simulink model "m03_model_for_HInf"  (R2021a)
settings: Solver=VariableStepAuto  StartTime=0.0  StopTime=20  MaxStep=1e-3  RelTol=1e-3
PreLoadFcn:
  | load feedforward_controller
InitFcn:
  | load feedforward_controller
libraries: cstblocks x3, acolibjan22 x3
settings Model: Creator=e102261  LastModifiedBy=jason
settings SolverCC: AlgebraicLoopSolver=TrustRegion
settings DataIOCC: SaveOutput=off  SignalLogging=off  DSMLogging=off  SaveTime=off  ReturnWorkspaceOutputs=off
settings DebuggingCC: ArithmeticOperatorsInVariantConditions=warning
settings SFSimCC: CustomCodeUndefinedFunction=UseInterfaceOnly

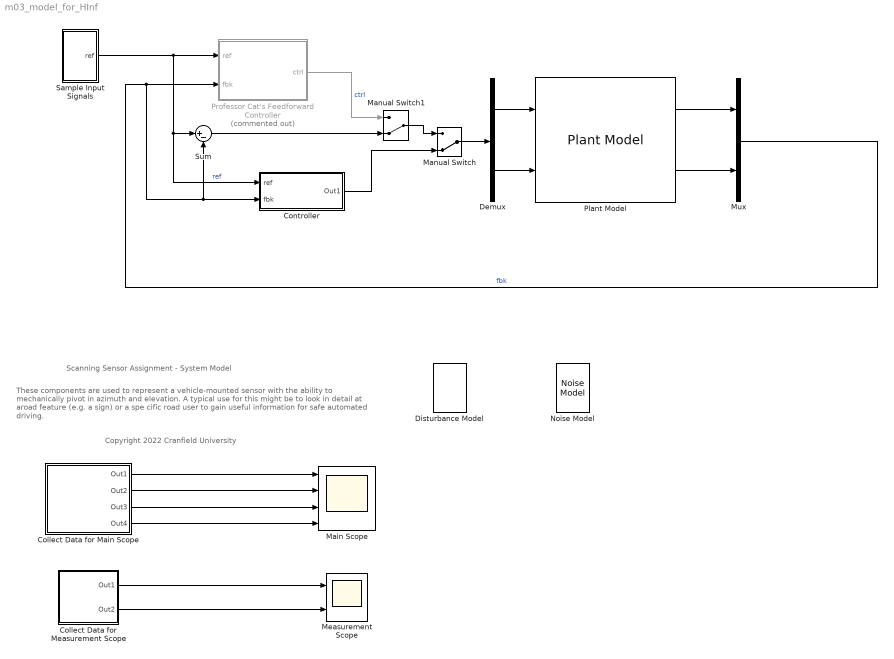
== system m03_model_for_HInf ==
  note: These components are used to represent a vehicle-mounted sensor with the ability to mechanically pivot in azimuth and elevation.  A typical use for this might be to look in
      | detail at aroad feature (e.g. a sign) or a spe cific road user to gain useful information for
      | safe automated driving.
  note: Scanning Sensor Assignment - System Model
  note: Copyright 2022 Cranfield University
  Collect Data for Main Scope : Subsystem
  Collect Data for Measurement Scope : Subsystem
  Controller : Subsystem
  Demux : Demux  Outputs=2
  Disturbance Model : acolibjan22/Disturbance Model  EnabledState=on
      settings: AttributesFormatString=|
      | Your control system is expected to
      | work with this enabled, but it is
      | sometimes helpful to turn it off for
      | debugging.
  Main Scope : Scope  NumInputPorts=4
  Manual Switch : ManualSwitch  CurrentSetting=0
  Manual Switch1 : ManualSwitch  CurrentSetting=0
  Measurement Scope : Scope  NumInputPorts=2
      settings: AttributesFormatString=|
      | There is nothing feedback control
      | can do to make these signals less
      | noisy, but you can reduce the amount
      | of this noise that gets fed back into
      | the control signals.
  Mux : Mux  Inputs=2
  Noise Model : acolibjan22/Noise Model  EnabledState=on
      settings: AttributesFormatString=|
      | Your control system is expected to
      | work with this enabled, but it is
      | sometimes helpful to turn it off for
      | debugging.
  Plant Model : acolibjan22/Plant Model  X0=0
  Professor Cat's Feedforward Controller : Subsystem  Commented=on  LoadFcn=load feedforward_controller  InitFcn=load feedforward_controller
      settings: AttributesFormatString=Your controller replaces this!
      mask Display: image('graphic1.jpg')
  Sample Input Signals : Subsystem
  Sum : Sum  Inputs=|+-
  wires:
  Plant Model/1 -> Mux/1
  Collect Data for Main Scope/1(Out1) -> Main Scope/1
  Collect Data for Main Scope/2(Out2) -> Main Scope/2
  Collect Data for Main Scope/3(Out3) -> Main Scope/3
  Collect Data for Main Scope/4(Out4) -> Main Scope/4
  Mux/1 -> Controller/2(fbk), Sum/2, Professor Cat's Feedforward Controller/2(fbk)  "fbk"
  Plant Model/2 -> Mux/2
  Demux/2 -> Plant Model/2
  Demux/1 -> Plant Model/1
  Collect Data for Measurement Scope/1(Out1) -> Measurement Scope/1
  Collect Data for Measurement Scope/2(Out2) -> Measurement Scope/2
  Sample Input Signals/1(ref) -> Sum/1, Controller/1(ref), Professor Cat's Feedforward Controller/1(ref)  "ref"
  Professor Cat's Feedforward Controller/1(ctrl) -> Manual Switch1/1  "ctrl"
  Manual Switch/1 -> Demux/1
  Controller/1(Out1) -> Manual Switch/2
  Sum/1 -> Manual Switch1/2
  Manual Switch1/1 -> Manual Switch/1

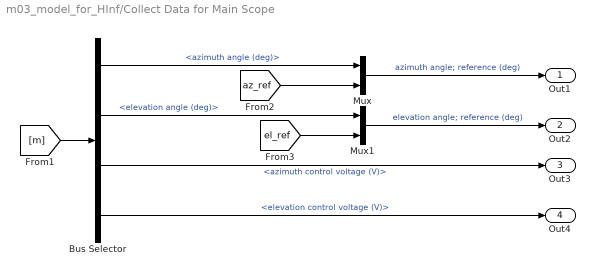
== system m03_model_for_HInf/Collect Data for Main Scope ==
  Bus Selector : BusSelector  OutputSignals=azimuth angle (deg),elevation angle (deg),azimuth control voltage (V),elevation control voltage (V)
  Mux : Mux  Inputs=2
  Mux1 : Mux  Inputs=2
  Out1 : Outport
  Out2 : Outport  Port=2
  Out3 : Outport  Port=3
  Out4 : Outport  Port=4
  wires:
  [m] -> Bus Selector/1
  Mux/1 -> Out1/1  "azimuth angle; reference (deg)"
  Bus Selector/1 -> Mux/1  "<azimuth angle (deg)>"
  [az_ref] -> Mux/2
  Bus Selector/2 -> Mux1/1  "<elevation angle (deg)>"
  [el_ref] -> Mux1/2
  Mux1/1 -> Out2/1  "elevation angle; reference (deg)"
  Bus Selector/3 -> Out3/1  "<azimuth control voltage (V)>"
  Bus Selector/4 -> Out4/1  "<elevation control voltage (V)>"

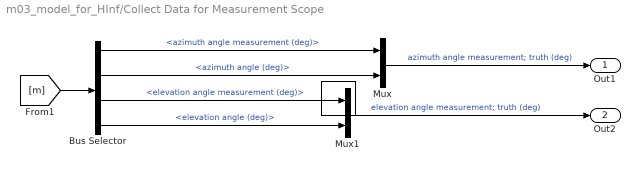
== system m03_model_for_HInf/Collect Data for Measurement Scope ==
  Bus Selector : BusSelector  OutputSignals=azimuth angle measurement (deg),azimuth angle (deg),elevation angle measurement (deg),elevation angle (deg)
  Mux : Mux  Inputs=2
  Mux1 : Mux  Inputs=2
  Out1 : Outport
  Out2 : Outport  Port=2
  wires:
  Mux1/1 -> Out2/1  "elevation angle measurement; truth (deg)"
  Bus Selector/4 -> Mux1/2  "<elevation angle (deg)>"
  Bus Selector/2 -> Mux/2  "<azimuth angle (deg)>"
  Mux/1 -> Out1/1  "azimuth angle measurement; truth (deg)"
  [m] -> Bus Selector/1
  Bus Selector/1 -> Mux/1  "<azimuth angle measurement (deg)>"
  Bus Selector/3 -> Mux1/1  "<elevation angle measurement (deg)>"

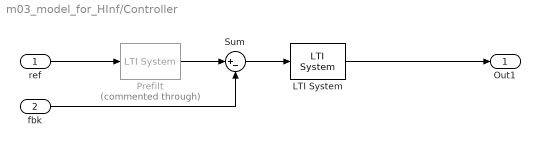
== system m03_model_for_HInf/Controller ==
  ref : Inport
  fbk : Inport  Port=2
  LTI System : cstblocks/LTI System  sys=C  IC=[]
  Prefilt : cstblocks/LTI System  Commented=through  sys=1  IC=[]
  Sum : Sum  Inputs=|+-
  Out1 : Outport
  wires:
  ref/1 -> Prefilt/1
  LTI System/1 -> Out1/1
  fbk/1 -> Sum/2
  Sum/1 -> LTI System/1
  Prefilt/1 -> Sum/1

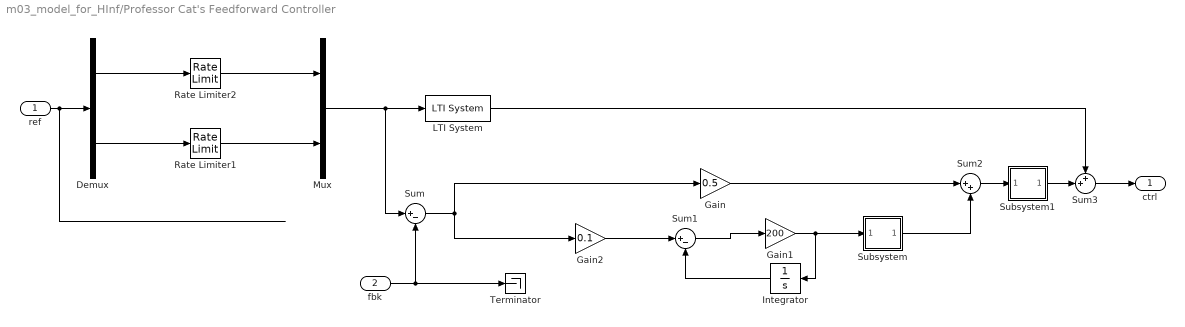
== system m03_model_for_HInf/Professor Cat's Feedforward Controller ==
  ref : Inport
  fbk : Inport  Port=2
  Demux : Demux  Outputs=2
  Gain : Gain  Gain=0.5
  Gain1 : Gain  Gain=200
  Gain2 : Gain  Gain=0.1
  Integrator : Integrator
  LTI System : cstblocks/LTI System  sys=Qff  IC=[]
      settings: AttributesFormatString=|
      | This is a feedforward controller
      | which tries to invert out any
      | unwanted dynamics and replaces
      | them with the ones we do want.
  Mux : Mux  Inputs=2
  Rate Limiter1 : RateLimiter  RisingSlewLimit=55  FallingSlewLimit=-55
      settings: AttributesFormatString=|
      | RisingSlewLimit=%<RisingSlewLimit>
      | FallingSlewLimit=%<FallingSlewLimit>
      | 
      | Professor Cat found that these limits were
      | needed to make his feedforward controller
      | work at all.  Why?
      | 
      | Can you manage without them with feedback?
      | Can they still be helpful with feedback?
      | There isn't a unique answer here.
  Rate Limiter2 : RateLimiter  RisingSlewLimit=55  FallingSlewLimit=-55
      settings: AttributesFormatString=|
      | RisingSlewLimit=%<RisingSlewLimit>
      | FallingSlewLimit=%<FallingSlewLimit>
  Subsystem : Subsystem
  Subsystem1 : Subsystem
  Sum : Sum  Inputs=|+-
  Sum1 : Sum  Inputs=|+-
  Sum2 : Sum  Inputs=|++
  Sum3 : Sum  Inputs=++|
  Terminator : Terminator
      settings: AttributesFormatString=|
      | Professor Cat doesn't know about feedback
      | control so he has ignored the feedback signal.
      | Don't do this! :-)
  ctrl : Outport
  wires:
  fbk/1 -> Sum/2, Terminator/1
  LTI System/1 -> Sum3/1
  Demux/1 -> Rate Limiter2/1
  Mux/1 -> Sum/1, LTI System/1
  Demux/2 -> Rate Limiter1/1
  Rate Limiter2/1 -> Mux/1
  Rate Limiter1/1 -> Mux/2
  ref/1 -> Demux/1
  Sum/1 -> Gain2/1, Gain/1
  Gain/1 -> Sum2/1
  Gain1/1 -> Subsystem/1(In1), Integrator/1
  Integrator/1 -> Sum1/2
  Sum1/1 -> Gain1/1
  Sum2/1 -> Subsystem1/1(In1)
  Gain2/1 -> Sum1/1
  Subsystem/1(Out1) -> Sum2/2
  Subsystem1/1(ctrl) -> Sum3/2
  Sum3/1 -> ctrl/1

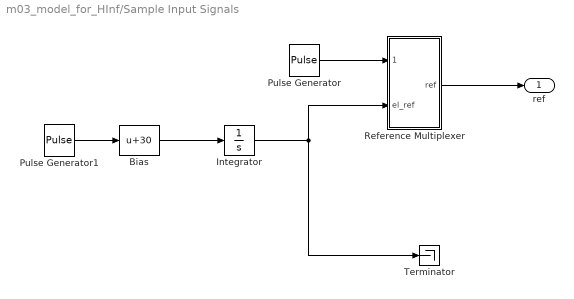
== system m03_model_for_HInf/Sample Input Signals ==
  Bias : Bias  Bias=30
  Integrator : Integrator
  Pulse Generator : DiscretePulseGenerator  PulseType=Time based  Amplitude=35  Period=10  PulseWidth=50  PhaseDelay=1
  Pulse Generator1 : DiscretePulseGenerator  PulseType=Time based  Amplitude=-120/2  Period=4  PulseWidth=50  PhaseDelay=2
  Reference Multiplexer : Subsystem
      settings: AttributesFormatString=|
      | Contains global GOTO
      | blocks for logging
  Terminator : Terminator
      settings: AttributesFormatString=|
      | This is the elevation velocity
      | if you need it for state space
      | control setpoints.
  ref : Outport
  wires:
  Pulse Generator/1 -> Reference Multiplexer/1(az_ref)
  Reference Multiplexer/1(ref) -> ref/1
  Integrator/1 -> Terminator/1, Reference Multiplexer/2(el_ref)
  Pulse Generator1/1 -> Bias/1
  Bias/1 -> Integrator/1

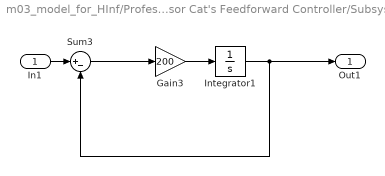
== system m03_model_for_HInf/Professor Cat's Feedforward Controller/Subsystem ==
  In1 : Inport
  Gain3 : Gain  Gain=200
  Integrator1 : Integrator
  Sum3 : Sum  Inputs=|+-
  Out1 : Outport
  wires:
  Integrator1/1 -> Out1/1, Sum3/2
  Gain3/1 -> Integrator1/1
  Sum3/1 -> Gain3/1
  In1/1 -> Sum3/1

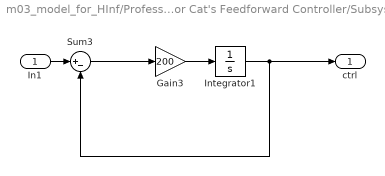
== system m03_model_for_HInf/Professor Cat's Feedforward Controller/Subsystem1 ==
  In1 : Inport
  Gain3 : Gain  Gain=200
  Integrator1 : Integrator
  Sum3 : Sum  Inputs=|+-
  ctrl : Outport
  wires:
  In1/1 -> Sum3/1
  Sum3/1 -> Gain3/1
  Gain3/1 -> Integrator1/1
  Integrator1/1 -> Sum3/2, ctrl/1

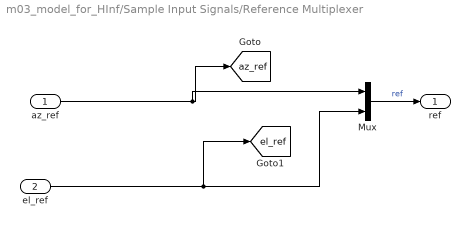
== system m03_model_for_HInf/Sample Input Signals/Reference Multiplexer ==
  az_ref : Inport
  el_ref : Inport  Port=2
  Mux : Mux  Inputs=2
  ref : Outport
  tag scope: az_ref=global, el_ref=global
  wires:
  Mux/1 -> ref/1  "ref"
  az_ref/1 -> Mux/1, [az_ref]
  el_ref/1 -> Mux/2, [el_ref]
